simulink library "lib_Encoder"  (R2018b)
settings: Solver=VariableStepAuto  StartTime=0.0  StopTime=10.0  RelTol=1e-3
settings Model: Creator=m.hiepp  LastModifiedBy=m.hiepp

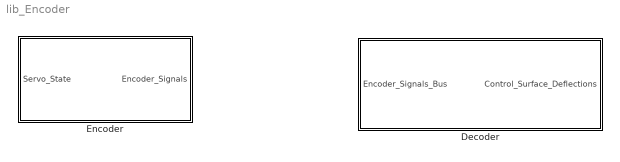
== system lib_Encoder ==
  Decoder : Subsystem
  Encoder : Subsystem

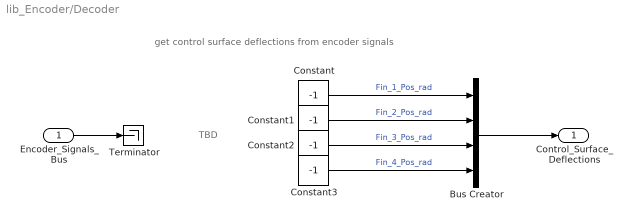
== system lib_Encoder/Decoder ==
  note: TBD
  note: get control surface deflections from encoder signals
  Encoder_Signals_Bus : Inport  OutDataTypeStr=Bus: Control_Surface_Encoder_Bus
  Bus Creator : BusCreator  Inputs=4  OutDataTypeStr=Bus: Control_Surface_Deflections_Bus
  Constant{,1..3} (4 alike) : Constant  Value=-1
  Terminator : Terminator
  Control_Surface_Deflections : Outport  OutDataTypeStr=Bus: Control_Surface_Deflections_Bus
  wires:
  Bus Creator/1 -> Control_Surface_Deflections/1
  Constant/1 -> Bus Creator/1  "Fin_1_Pos_rad"
  Constant1/1 -> Bus Creator/2  "Fin_2_Pos_rad"
  Constant2/1 -> Bus Creator/3  "Fin_3_Pos_rad"
  Constant3/1 -> Bus Creator/4  "Fin_4_Pos_rad"
  Encoder_Signals_Bus/1 -> Terminator/1

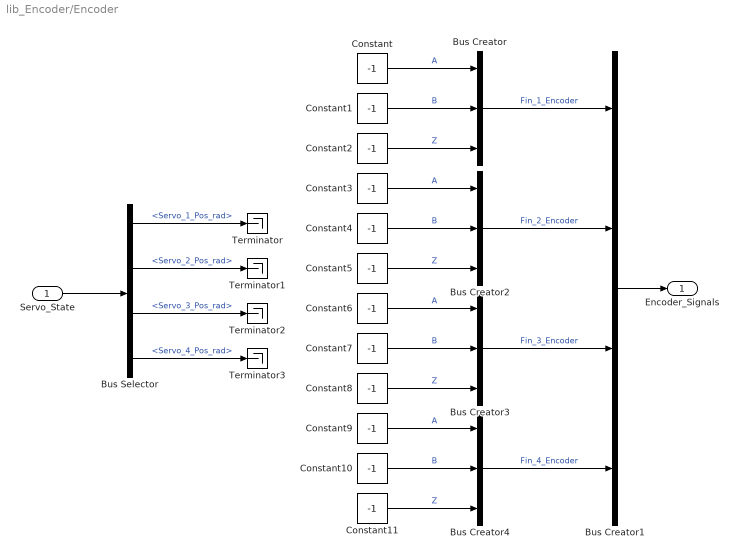
== system lib_Encoder/Encoder ==
  Servo_State : Inport  OutDataTypeStr=Bus: Servo_State_Bus
  Bus Creator{,2..4} (4 alike) : BusCreator  Inputs=3  OutDataTypeStr=Bus: Inc_Encoder_Signal_Bus
  Bus Creator1 : BusCreator  Inputs=4  OutDataTypeStr=Bus: Control_Surface_Encoder_Bus
  Bus Selector : BusSelector  OutputSignals=Servo_Positions.Servo_1_Pos_rad,Servo_Positions.Servo_2_Pos_rad,Servo_Positions.Servo_3_Pos_rad,Servo_Positions.Servo_4_Pos_rad
  Constant{,1..11} (12 alike) : Constant  Value=-1
  Terminator{,1..3} (4 alike) : Terminator
  Encoder_Signals : Outport  OutDataTypeStr=Bus: Control_Surface_Encoder_Bus
  wires:
  Bus Creator1/1 -> Encoder_Signals/1
  Servo_State/1 -> Bus Selector/1
  Bus Creator/1 -> Bus Creator1/1  "Fin_1_Encoder"
  Bus Creator4/1 -> Bus Creator1/4  "Fin_4_Encoder"
  Bus Creator3/1 -> Bus Creator1/3  "Fin_3_Encoder"
  Bus Creator2/1 -> Bus Creator1/2  "Fin_2_Encoder"
  Bus Selector/1 -> Terminator/1  "<Servo_1_Pos_rad>"
  Bus Selector/4 -> Terminator3/1  "<Servo_4_Pos_rad>"
  Bus Selector/3 -> Terminator2/1  "<Servo_3_Pos_rad>"
  Bus Selector/2 -> Terminator1/1  "<Servo_2_Pos_rad>"
  Constant/1 -> Bus Creator/1  "A"
  Constant11/1 -> Bus Creator4/3  "Z"
  Constant10/1 -> Bus Creator4/2  "B"
  Constant9/1 -> Bus Creator4/1  "A"
  Constant8/1 -> Bus Creator3/3  "Z"
  Constant7/1 -> Bus Creator3/2  "B"
  Constant6/1 -> Bus Creator3/1  "A"
  Constant5/1 -> Bus Creator2/3  "Z"
  Constant4/1 -> Bus Creator2/2  "B"
  Constant3/1 -> Bus Creator2/1  "A"
  Constant2/1 -> Bus Creator/3  "Z"
  Constant1/1 -> Bus Creator/2  "B"
